simulink model "ee145L3p4"  (R2019a)
settings: Solver=VariableStepAuto  StartTime=0.0  StopTime=10.0  RelTol=1e-3
values from neighbouring files (symbols this model uses):
  A = [k1 0 0;0 0 V; 0 k2 k3]    [ss_inputsL3.m]
  B = [1 0; 0 0; 0 1]    [ss_inputsL3.m]
  C = [1 0 0; 0 1 0; 0 0 1]    [ss_inputsL3.m]
  D = [0, 0; 0, 0; 0, 0]    [ss_inputsL3.m]
settings Model: OrderedModelArguments=off  Creator=sk  LastModifiedBy=sk

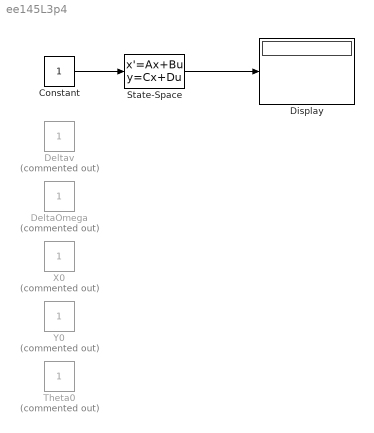
== system ee145L3p4 ==
  Constant : Constant
  DeltaOmega : Constant  Commented=on
  Deltav : Constant  Commented=on
  Display : Display
  State-Space : StateSpace  A=A  B=B  C=C  D=D  InitialCondition=0  ContinuousStateAttributes="''unicycle\""
  Theta0 : Constant  Commented=on
  X0 : Constant  Commented=on
  Y0 : Constant  Commented=on
  wires:
  Constant/1 -> State-Space/1
  State-Space/1 -> Display/1
